simulink model "P3P_Grunert"  (R2023b)
settings: Solver=FixedStepDiscrete  StartTime=0.0  StopTime=0  RelTol=1e-3
values from neighbouring files (symbols this model uses):
  checkerSize = [5, 8]    [P3P_processVideo.m]
  checkerSquareLength = 31    [P3P_processVideo.m]
  I_current = I_allFrames(:,:,q)    [P3P_processVideo.m]
  K = [1109 0 640; 0 1109 360; 0 0 1]    [P3P_processVideo.m]
  x_pnts_i = round(x_pnts_i)    [P3P_processVideo.m]
  X_pnts_w = calcCheckerEdgeCoords_w(checkerSize, checkerSquareLength)    [P3P_processVideo.m]
undefined symbols (not defined in the file or in its folder): gray, Rec, SDTV
libraries: dspinverses x5, dspmathops x5, visiontextngfix x4, matrix_library x2, visionconversions x1, visionanalysis x1, dspvision x1, visionsources x1
(part 3 of 3)

== matlab function P3P_Grunert/Subsystem/Custom P3P solver (Grunert)/Find ray lengths jingnanshi convention ==
  data: l_AB input; soln output size=[8, 3]; l_BC input; l_AC input; theta input
function soln = fcn(l_AB, l_BC, l_AC, theta)

soln = zeros(8, 3);


%Calculate polynomial coefficients
a = l_AC;
b = l_BC;
c = l_AB;

gamma = theta(1); %theta_AB
alpha = theta(3); %theta_AC
beta = theta(2); %theta_BC


a2minc2ovb2 =  (a^2 - c^2) / b^2 ;
a2plusc2ovb2 =  (a^2 + c^2) / b^2; 


A0 = (1 + a2minc2ovb2)^2   -   4*((a*cos(gamma)/b)^2);
A1 = - a2minc2ovb2 * (1 + a2minc2ovb2) * cos(beta)     +    2 * ((a * cos(gamma) /  b)^2) * cos (beta)     -     (1 - a2plusc2ovb2) * cos(alpha) * cos(gamma);
A1 = 4 * A1;
A2 = a2minc2ovb2^2   -   1   +   2*((a2minc2ovb2 * cos(beta))^2)  +  2 *(  ((b^2 - c^2)/(b^2))  * (cos(alpha))^2  )   - 4*a2plusc2ovb2*cos(alpha)*cos(beta)*cos(gamma)   +   2*((b^2 - a^2)/(b^2))*((cos(gamma))^2);
A2 = 2* A2;
A3 = a2minc2ovb2 * (1 - a2minc2ovb2) * cos(beta)    -   (1 - a2plusc2ovb2) * cos(alpha) * cos(gamma)    +   2 * ((c * cos(alpha)/b)^2) * cos(beta);
A3 = 4 * A3;
A4 = (a2minc2ovb2 -1)^2   - (2 * c * cos(alpha) / b)^2;

%Solve polynomial
%instead of u and v for polynomial, use g and h - i.e., g = s2/s1 and h =
%s3/s1
p = [A4 A3 A2 A1 A0];
h = roots(p);
%choose only real roots - maybe this is not necessary?
h = h(imag(h)==0);
h = real(h);

%%%%%%%%%%%%%%%%%%%%%%%%%%%%%%%%%%%%%%%%%
%%%%%%%%%%%%%Find ray lengths

%For s1, which corresponds to sB. Should end up with 4 solns
%s_A =    (b^2) / (1 + h.^2  +  2*h*cos(beta)  )     ;
%s_A = s_A(s_A~=0);
%s_A = transpose(s_A);
%s_A = s_A.^0.5;


%Find s2, which corresponds to sC.
counter = 1;
for i = 1:numel(h)

    s_1 = (b^2) / (1 + (h(i)^2) - 2*h(i)*cos(beta));
    s_1 = sqrt(s_1);

    G2 = s_1^2;
    G1 = - 2 * (s_1^2) * cos(gamma);
    G0 = (s_1^2 -c^2);

    g = roots([G2 G1 G0]);
    g = g(imag(g)==0);
    g = real(g);

    %First, solve for s_C, since it only depends on h and s_A:

    for j = 1:numel(g)
        soln(counter, 1) = s_1 * g(j);
        soln(counter, 3) = s_1 * h(i);
        soln(counter, 2) = s_1; 
        counter = counter +1;
    end

end

== matlab function P3P_Grunert/Subsystem/Custom P3P solver (Grunert)/MATLAB Function4 ==
  data: pnts_vectorsCameraCoords input; theta_raysABC_radians output
function theta_raysABC_radians = calcProjectionRayAngles(pnts_vectorsCameraCoords)

A_x_c = pnts_vectorsCameraCoords(:,1);
B_x_c = pnts_vectorsCameraCoords(:,2);
C_x_c = pnts_vectorsCameraCoords(:,3);

%theta_AB = acos(dot(A_x_c, B_x_c));
%theta_BC = acos(dot(B_x_c, C_x_c));
%theta_AC = acos(dot(C_x_c, A_x_c));

%theta_AB = atan2(norm(cross(A_x_c, B_x_c)), dot(A_x_c, B_x_c));
%theta_BC = atan2(norm(cross(B_x_c, C_x_c)), dot(B_x_c, C_x_c));
%theta_AC = atan2(norm(cross(A_x_c, C_x_c)), dot(A_x_c, C_x_c)); 

theta_AB = acos(dot(A_x_c, B_x_c)/(norm(A_x_c)*norm(B_x_c)));
theta_BC = acos(dot(B_x_c, C_x_c)/(norm(B_x_c)*norm(C_x_c)));
theta_AC = acos(dot(A_x_c, C_x_c)/(norm(A_x_c)*norm(C_x_c)));


theta_raysABC_radians = [theta_AB; theta_BC; theta_AC];

== matlab function P3P_Grunert/MATLAB Function ==
  data: checkerSize input; X_pts_w output size=[60,3]; squareEdgeLength input
function X_pts_w = calcCheckerEdgeCoords_w(checkerSize, squareEdgeLength)
    
    boardWidth = checkerSize(2);
    boardHeight = checkerSize(1);
    X_pts_w = zeros((boardWidth-1)*(boardHeight-1), 3);

    %for each column
    for c=1 : boardWidth-1
        for r = 1: boardHeight-1
            x = (c-1)*squareEdgeLength;
            y = (r-1)*squareEdgeLength;
            z = 0;
            X_pts_w(  (((c-1)*(boardHeight-1)) + r), 1) = x;
            X_pts_w(  (((c-1)*(boardHeight-1)) + r), 2) = y;
            X_pts_w(  (((c-1)*(boardHeight-1)) + r), 3) = z;
        end
    end
end

== matlab function P3P_Grunert/Subsystem/Custom P3P solver (Kneip)/Gao P3P by Nagano ==
  data: f_unitVecs input; Rt_C_W output size=[3,4,4]; X_ABC_W input
function Rt_C_W = fcn(f_unitVecs, X_ABC_W)

Rt_C_W = zeros(3,4,4);

coder.extrinsic('p3p_gao');
[R, t] = p3p_gao(f_unitVecs, X_ABC_W);
Rt_C_W(1:3,1:3,1:4)=R(1:3,1:3,1:4);
for i=1:4
    Rt_C_W(1:3,4,i)=t(1:3,i);
end

== matlab function P3P_Grunert/Subsystem/Custom P3P solver (Kneip)/MATLAB Function ==
  data: f_unitVecs input; Rt_C_W output size=[3,4,4]; X_ABC_W input; Rt_W_C output
function [Rt_C_W, Rt_W_C]= fcn(f_unitVecs, X_ABC_W)

%Kneip's parametrization of P3P. 
%Let P1 = A, P2 = B, P3 = C. Let cam centre be P. Thus, beta = L(APB);
%alpha = L(BAP). Also, the vectors f1 = fA, f2 = fB, f3 = fC. Nu is camera
%frame, tau is intermediate camera frame. 


%% Assign some variables
f1 = f_unitVecs(:,1);
f2 = f_unitVecs(:,2);
f3 = f_unitVecs(:,3);
P1 = X_ABC_W(:,1);
P2 = X_ABC_W(:,2);
P3 = X_ABC_W(:,3);


%% Define intermediate frame Tau
tau_x = f1;
tau_z = cross(f1, f2);
tau_z = tau_z/norm(tau_z); %normalise
tau_y = cross(tau_z, tau_x);
T_tau_nu = [tau_x tau_y tau_z]; %Rotation matrix
T_nu_tau = transpose(T_tau_nu);%Transform from cam frame nu to intermed frame tau (no translation)

%% Define intermediate world frame Eta
P1P2 = P2-P1;
P1P3 = P3-P1;
d12 = norm(P1P2); %More efficient to calculate here
eta_x = P1P2/d12;
eta_z = cross(eta_x, P1P3);
eta_z = eta_z/norm(eta_z); %normalise
eta_y = cross(eta_z, eta_x);
T_eta_W = [eta_x eta_y eta_z];
T_W_eta = transpose(T_eta_W); %Transform from world to eta

%% Calculate constants
%Convert vector f3 into frame tau (needed for phi calc)
f3_tau = T_nu_tau * f3;

%Convert P3 into frame eta (needed for p1, p2 calc)
P3_eta = T_W_eta * (P3 - P1);


%Calculate beta, i.e., L(APB)
cosBeta = dot(f1, f2);

% Calculate constants
b = sqrt((1/(1-cosBeta^2))-1);
if cosBeta < 0
    b = -b;
end

phi1 = f3_tau(1)/f3_tau(3); %x/z
phi2 = f3_tau(2)/f3_tau(3); %y/z

p1 = P3_eta(1);
p2 = P3_eta(2);

%d12 calculated earlier

%% Set up quartic terms

a4 = -(phi2^2)*(p2^4) - (phi1^2)*(p2^4) - (p2^4);
a3 = 2*(p2^3)*d12*b  +  2*(phi2^2)*(p2^3)*d12*b  -  2*phi1*phi2*(p2^3)*d12;
a2 = -(phi2*p1*p2)^2  -  phi2*(p2*d12*b)^2  -  (phi2*p2*d12)^2  +  (phi2*p2)^2  +  (phi1^2)*(p2^4)  +  2*p1*(p2^2)*d12  +  2*phi1*phi2+p1*(p2^2)*d12*b  -  (phi1*p1*p2)^2  +  2*(phi2^2)*p1*(p2^2)*d12  -  (p2*d12*b)^2  -  2*(p1*p2)^2;
a1 = 2*(p1^2)*p2*d12*b  +  2*phi1*phi2*(p2^3)*d12  -  2*(phi2^2)*(p2^3)*d12*b  -  2*p1*p2*(d12^2)*b;
a0 = -2*phi1*phi2*p1*(p2^2)*d12*b  +  (phi2*p2*d12)^2  +  2*(p1^3)*d12  -  (p1*d12)^2  +  (phi2*p1*p2)^2  -  (p1^4)  -  2*(phi2^2)*p1*(p2^2)*d12  +  (phi1*p1*p2)^2  +  (phi2*p2*d12*b)^2;


%% Solve quartic to find cosTheta
q = [a4 a3 a2 a1 a0];
cosTheta = roots(q);
cosTheta = real(cosTheta);

%% Subst. to find cotAlpha
cotAlpha = zeros(4);

num = ((phi1*p1)/phi2) - (d12*b);
den = (d12 - p1);
for i = 1:numel(cosTheta)
    cotAlpha(i) = (num + p2*cosTheta(i))/(den + (phi1*p2/phi2)*cosTheta(i));
end

%% Extract angles
alpha = zeros(4);
theta = zeros(4);
sinTheta = zeros(4);
sinAlpha = zeros(4);
cosAlpha = zeros(4);
for i = 1:numel(cosTheta)

    sinTheta(i) = sqrt(1-(cosTheta(i)^2));
    sinAlpha(i) = sqrt(1/((cotAlpha(i)^2)+1));
    cosAlpha(i) = sqrt(1-(sinAlpha(i)^2));

    %Apply angle conditions
    if f3_tau(3)>0
        sinTheta(i) = -sinTheta(i);
    end
    if cotAlpha(i)<0
        cosAlpha(i) = -cosAlpha(i);
    end
    
end

%% Subst. angles to find position of camera centre P inside int. frame Eta
P_eta = zeros(3,4);
for i = 1:numel(cosTheta)
    P_eta(1,i) = d12 * cosAlpha(i) * ((b*sinAlpha(i))+cosAlpha(i));
    P_eta(2,i) = d12 * sinAlpha(i) * cosTheta(i) * ((b*sinAlpha(i))+cosAlpha(i));
    P_eta(3,i) = d12 * sinAlpha(i) * sinTheta(i) * ((b*sinAlpha(i))+cosAlpha(i));
end

%% Subst angles to find transformation from Eta to Tau
T_eta_tau = zeros(3,3,4);
for i = 1:numel(cosTheta)
    T_eta_tau(:,1,i) = [-cosAlpha(i), sinAlpha(i), 0];
    T_eta_tau(:,2,i) = [-sinAlpha(i)*cosTheta(i), -cosAlpha(i)*cosTheta(i), -sinTheta(i)];
    T_eta_tau(:,3,i) = [-sinAlpha(i)*sinTheta(i), -cosAlpha(i)*sinTheta(i), cosTheta(i)];
end

%% Now we have everything we need! 
%Calculater translation vectors
translation_C_W = zeros(3,4);
rot_C_W = zeros(3,3,4);
Rt_C_W = zeros(3,4,4);
Rt_W_C = zeros(3,4,4);
for i = 1:numel(cosTheta)
    translation_C_W(:,i) = P1 + T_eta_W * P_eta(:,i);
    rot_C_W(:,:,i) =  T_eta_W * transpose(T_eta_tau(:,:,i)) * T_nu_tau;
    
    Rt_C_W(1:3,1:3,i) = rot_C_W(1:3,1:3,i);
    Rt_C_W(1:3,4,i) = translation_C_W(1:3,i);

    %Calc inverse, in case
    Rt_W_C(1:3,1:3,i) = transpose(Rt_C_W(1:3,1:3,i));
    Rt_W_C(1:3,4,i) = - Rt_W_C(1:3,1:3,i)*translation_C_W(1:3,i);

end

%% Do some plotting for verification
%coder.extrinsic('verifyKneipCoordSys');
%verifyKneipCoordSys(T_nu_tau, T_W_eta);
